simulink model "DroneAttitudeSim1"  (R2023b)
settings: Solver=VariableStepAuto  StartTime=0.0  StopTime=15  RelTol=1e-3
values from neighbouring files (symbols this model uses):
  G = [0 0 0 0]'    [DroneAttitude1.m]
  I_x = 3.88 * 10^-2    (= 0.0388)    [DroneAttitude1.m]
  I_y = 3.87 * 10^-2    (= 0.0387)    [DroneAttitude1.m]
  I_z = 1.15 * 10^-3    (= 0.00115)    [DroneAttitude1.m]
undefined symbols (not defined in the file or in its folder): K
libraries: shared6dof x1
settings Model: Creator=jacksonwright  LastModifiedBy=jacksonwright

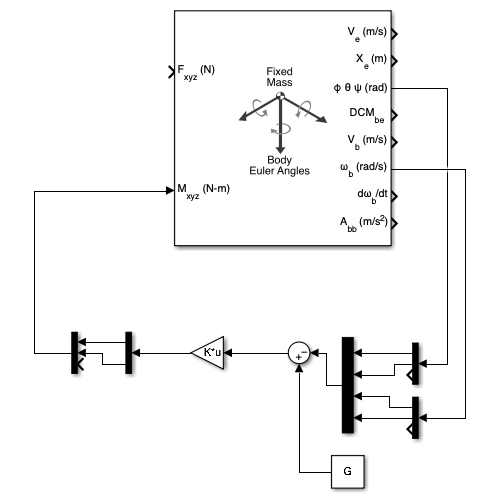
[thumbnail: Simulink's stored preview of the top-level diagram]
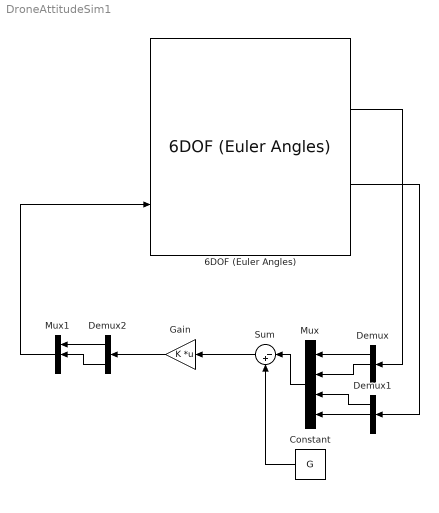
== system DroneAttitudeSim1 ==
  6DOF (Euler Angles) : shared6dof/6DOF (Euler Angles)  units=Metric (MKS)  mtype=Fixed  rep=Euler Angles  xme_0=[0 0 0]  Vm_0=[0 0 0]  eul_0=[0.5 0 0]  pm_0=[0 0 0]  mass_0=1.0  mass_e=0.5  mass_f=2.0  inertia=diag([I_x,I_y, I_z])  inertia_e=eye(3)  inertia_f=2*eye(3)  k_quat=1.0  vre_flag=on  abi_flag=off  aMode=0  xme_statename=''  Vm_statename=''  eul_statename=''  quat_statename=''  pm_statename=''  mass_statename=''
  Constant : Constant  Value=G
  Demux : Demux  Outputs=3
  Demux1 : Demux  Outputs=3
  Demux2 : Demux  Outputs=2
  Gain : Gain  Gain=K  Multiplication=Matrix(K*u)
  Mux : Mux
  Mux1 : Mux  Inputs=3
  Sum : Sum  Inputs=|-+
  wires:
  Constant/1 -> Sum/2
  6DOF (Euler Angles)/3 -> Demux/1
  Demux/1 -> Mux/1
  Demux/2 -> Mux/2
  Mux/1 -> Sum/1
  Sum/1 -> Gain/1
  6DOF (Euler Angles)/6 -> Demux1/1
  Demux1/1 -> Mux/3
  Demux1/2 -> Mux/4
  Gain/1 -> Demux2/1
  Demux2/1 -> Mux1/1
  Demux2/2 -> Mux1/2
  Mux1/1 -> 6DOF (Euler Angles)/2
